simulink model "lqg_cartpend_sim_modified3"  (R2015a)
settings: Solver=ode45  StartTime=0.0  StopTime=10.0  RelTol=1e-3
values from neighbouring files (symbols this model uses):
  C = cos( y(:,3) )    [cartPendMatrix.m]    (also in cartPendVector.m = cos( y(3) ); run_cartPend_LQG.m = [1 1 1 1]; run_cartPend_kalmanFilter.m = [1 0 0 0]; run_cartPend_obs.m = [0 1 0 0])
  K = place(A, B, p )    [run_cartPend.m]    (also in run_cartPend_LQG.m = [0,0,0,0]; run_cartPend_LQR.m = lqr( A,B,Q,R); run_cartPend_linearizedControl.m; simulink_cartPend_initialize.m = [0,0,0,0])
  sysKF = ss(A-Lmat*C,[B Lmat],eye(4),0*[B Lmat])    [run_cartPend_LQG.m]    (also in run_cartPend_kalmanFilter.m = ss(A-Kf*C,[B Kf],eye(4),0*[B Kf]))
settings Model: Creator=Thomas  LastModifiedBy=Thomas

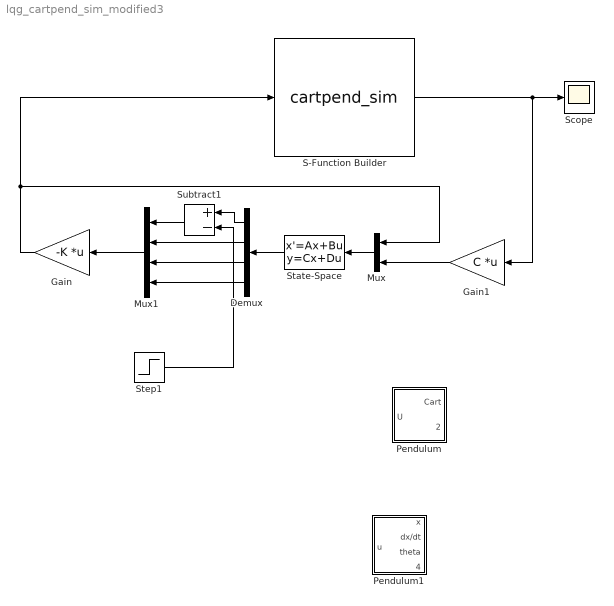
== system lqg_cartpend_sim_modified3 ==
  Demux : Demux
  Gain : Gain  Gain=-K  Multiplication=Matrix(K*u) (u vector)
  Gain1 : Gain  Gain=C  Multiplication=Matrix(K*u) (u vector)
  Mux : Mux  Inputs=2
  Mux1 : Mux
  Pendulum : Subsystem  mask(Inverted pendulum on cart){Mcart=0.455, m=0.21, l=0.61/2, g=9.8}
      mask prompts: Mcart "Mass of cart (kg):"; m "Mass of pendulum (kg):"; l "Distance to pendulum center of mass(m):"; g "Acceleration of gravity (m/s^2):"
      mask help: Unmask and double-click to see dynamics
      mask Help: Nonlinear dynamics of inverted pendulum on cart.
  Pendulum1 : Subsystem  mask(Inverted pendulum on cart){Mcart=0.455, m=0.21, l=0.61/2, g=9.8}
      mask prompts: Mcart "Mass of cart (kg):"; m "Mass of pendulum (kg):"; l "Distance to pendulum center of mass(m):"; g "Acceleration of gravity (m/s^2):"
      mask help: Unmask and double-click to see dynamics
      mask Help: Nonlinear dynamics of inverted pendulum on cart.
  S-Function Builder : S-Function  InitFcn=try, set_param(gcb,'FunctionName','cartpend_sim'), end  FunctionName=cartpend_sim  SFunctionModules=cartpend_sim_wrapper  mask(S-Function Builder){}
      mask help: Simulink:masks:SFunctionBuilder_MD
      mask init:
      | val = [[.9  0.75 0.75 1 1 .9 .9 1]',[1 1 0.75 0.75 .9 .9 1 .9]'];try , sys = get_param(gcb,'SfunBuilderFcnName');if isempty(sys), sys = get_param(gcb,'FunctionName'); end,catch, sys = get_param(gcb,'FunctionName'); end
      settings: CopyFcn=set_param(gcbh,'LinkStatus','none')  PreSaveFcn=try, set_param(gcb,'FunctionName','cartpend_sim'), end  OpenFcn=sfunctionwizard(gcbh)
      mask Display: plot(val(:,1),val(:,2)),disp(sys), port_label('input',1,'u0'), port_label('output',1,'y0')
  Scope : Scope
      settings: YMin=-0.59265  YMax=3.57093
  State-Space : StateSpace  A=sysKF.a  B=sysKF.b  C=sysKF.c  D=sysKF.d  X0=[0 0 0 0]
  Step1 : Step  Time=10  SampleTime=0
  Subtract1 : Sum  Inputs=+-
  wires:
  Gain/1 -> Mux/1, S-Function Builder/1
  S-Function Builder/1 -> Gain1/1, Scope/1
  Mux/1 -> State-Space/1
  Demux/2 -> Mux1/2
  Demux/4 -> Mux1/4
  Demux/3 -> Mux1/3
  Mux1/1 -> Gain/1
  Subtract1/1 -> Mux1/1
  Demux/1 -> Subtract1/1
  Step1/1 -> Subtract1/2
  State-Space/1 -> Demux/1
  Gain1/1 -> Mux/2

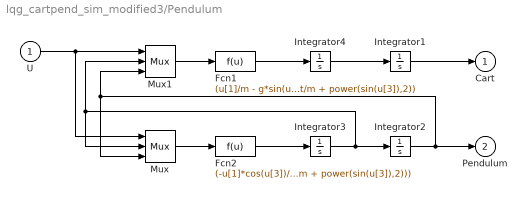
== system lqg_cartpend_sim_modified3/Pendulum ==
  U : Inport
  Fcn1 : Fcn  Expr=(u[1]/m - g*sin(u[3])*cos(u[3]) + l*power(u[2],2)*sin(u[3]))/(Mcart/m + power(sin(u[3]),2))
  Fcn2 : Fcn  Expr=(-u[1]*cos(u[3])/m + (Mcart+m)*g*sin(u[3])/m - l*power(u[2],2)*sin(u[3])*cos(u[3]))/(l*(Mcart/m + power(sin(u[3]),2)))
  Integrator{1..4} (4 alike) : Integrator
  Mux : Mux  Inputs=3
  Mux1 : Mux  Inputs=3
  Cart : Outport  InitialOutput=0
  Pendulum : Outport  Port=2  InitialOutput=0
  wires:
  Integrator1/1 -> Cart/1
  Fcn2/1 -> Integrator3/1
  Mux/1 -> Fcn2/1
  Mux1/1 -> Fcn1/1
  Fcn1/1 -> Integrator4/1
  Integrator4/1 -> Integrator1/1
  U/1 -> Mux1/1, Mux/1
  Integrator3/1 -> Integrator2/1, Mux1/2, Mux/2
  Integrator2/1 -> Pendulum/1, Mux1/3, Mux/3

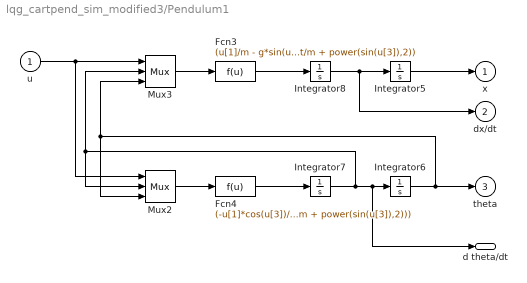
== system lqg_cartpend_sim_modified3/Pendulum1 ==
  u : Inport
  Fcn3 : Fcn  Expr=(u[1]/m - g*sin(u[3])*cos(u[3]) + l*power(u[2],2)*sin(u[3]))/(Mcart/m + power(sin(u[3]),2))
  Fcn4 : Fcn  Expr=(-u[1]*cos(u[3])/m + (Mcart+m)*g*sin(u[3])/m - l*power(u[2],2)*sin(u[3])*cos(u[3]))/(l*(Mcart/m + power(sin(u[3]),2)))
  Integrator{5..8} (4 alike) : Integrator
  Mux2 : Mux  Inputs=3
  Mux3 : Mux  Inputs=3
  x : Outport  InitialOutput=0
  dx/dt : Outport  Port=2  InitialOutput=0
  "theta " : Outport  Port=3  InitialOutput=0
  d theta/dt : Outport  Port=4  InitialOutput=0
  wires:
  Integrator5/1 -> x/1
  Fcn4/1 -> Integrator7/1
  Mux2/1 -> Fcn4/1
  Mux3/1 -> Fcn3/1
  Fcn3/1 -> Integrator8/1
  Integrator8/1 -> dx/dt/1, Integrator5/1
  u/1 -> Mux3/1, Mux2/1
  Integrator7/1 -> d theta/dt/1, Integrator6/1, Mux3/2, Mux2/2
  Integrator6/1 -> "theta "/1, Mux3/3, Mux2/3
